simulink model "state_machine_by_code"  (R2021b)
settings: Solver=ode4  StartTime=0.0  StopTime=inf  FixedStep=0.001  RelTol=1e-3  EnableMultiTasking=on
model workspace (MATLAB code in the model file):
  | addpath src\model
  | addpath src\utils
libraries: rtlab x2
Description:
  | Model of a simple control system for use iin training.
settings Model: Creator=Paul Baracos  LastModifiedBy=andrerangel
settings SolverCC: AlgebraicLoopSolver=TrustRegion
settings DataIOCC: LimitDataPoints=on  SaveFormat=Array  SignalLoggingSaveFormat=ModelDataLogs  SaveOutput=off  SaveTime=off  ReturnWorkspaceOutputs=off  SignalLoggingName=sigsOut
settings OptimizationCC: BlockReduction=off  BooleanDataType=off  OptimizeBlockIOStorage=off  BufferReuse=off  ExpressionFolding=off  LocalBlockOutputs=off  InitFltsAndDblsToZero=on  LifeSpan=inf
settings DebuggingCC: SaveWithParameterizedLinksMsg=none  UnderspecifiedInitializationDetection=Classic  MergeDetectMultiDrivingBlocksExec=none  SignalResolutionControl=TryResolveAllWithWarning  MultiTaskDSMMsg=warning  MultiTaskCondExecSysMsg=none  FcnCallInpInsideContextMsg=warning  SFUnexpectedBacktrackingDiag=warning  SFNoUnconditionalDefaultTransitionDiag=warning  SFExecutionAtInitializationDiag=none  SFMachineParentedDataDiag=warning  ArithmeticOperatorsInVariantConditions=warning
settings HardwareCC: ProdBitPerPointer=32  ProdBitPerSizeT=32  ProdBitPerPtrDiffT=32  ProdLargestAtomicFloat=None  ProdIntDivRoundTo=Undefined  ProdEndianess=Unspecified  ProdWordSize=32  ProdHWDeviceType=32-bit Generic  TargetUnknown=on
settings ModelReferenceCC: PropagateSignalLabelsOutOfModel=off
settings SFSimCC: SimUseLocalCustomCode=off  CustomCodeUndefinedFunction=UseInterfaceOnly
settings RTWCC: RTWUseLocalCustomCode=off
settings CodeAppCC: StateflowObjectComments=on
settings GRTTargetCC: TargetFcnLib=ansi_tfl_tmw.mat  TargetLangStandard=C89/C90 (ANSI)  CombineOutputUpdateFcns=off  GRTInterface=on
settings ConfigComp: CovMetricSettings=dw  CovSaveCumulativeToWorkspaceVar=on  CovSaveSingleToWorkspaceVar=on  CovExternalEMLEnable=off

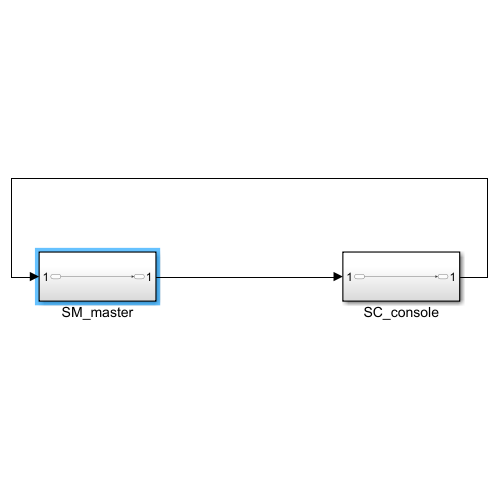
[thumbnail: Simulink's stored preview of the top-level diagram]
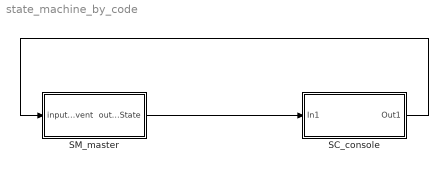
== system state_machine_by_code ==
  SC_console : Subsystem
  SM_master : Subsystem
  wires:
  SM_master/1(outputState) -> SC_console/1(In1)
  SC_console/1(Out1) -> SM_master/1(inputEvent)

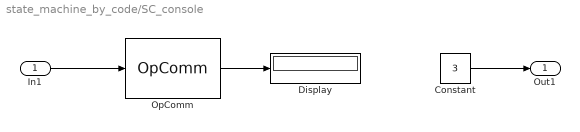
== system state_machine_by_code/SC_console ==
  In1 : Inport
  Constant : Constant  Value=3
  Display : Display
  OpComm : rtlab/OpComm  nbport=1  groupe_acq=1  subsys_rate=0  st=0  Synchronization=on  Interpolation=on  Threshold=1.0  Missed_Data=off  Sim_Time=off  Samples=off  dynSigOut=off  from_console=0  warning_done=off  writeOpCommFile=off  Offset=off
      settings: SourceProductName=RT-LAB
  Out1 : Outport
  wires:
  In1/1 -> OpComm/1
  Constant/1 -> Out1/1
  OpComm/1 -> Display/1

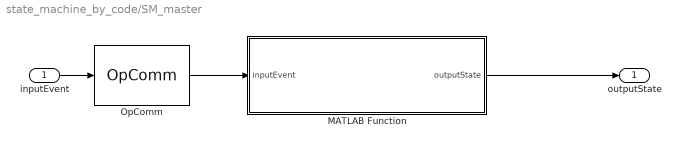
== system state_machine_by_code/SM_master ==
  inputEvent : Inport
  MATLAB Function : MATLAB Function  TreatAsAtomicUnit=on
  OpComm : rtlab/OpComm  nbport=1  groupe_acq=1  subsys_rate=0  st=0  Synchronization=on  Interpolation=on  Threshold=1.0  Missed_Data=off  Sim_Time=off  Samples=off  dynSigOut=off  from_console=1  warning_done=off  writeOpCommFile=off  Offset=off
      settings: SourceProductName=RT-LAB
  outputState : Outport
  wires:
  inputEvent/1 -> OpComm/1
  MATLAB Function/1(outputState) -> outputState/1
  OpComm/1 -> MATLAB Function/1(inputEvent)

== matlab function state_machine_by_code/SM_master/MATLAB Function ==
  data: inputEvent input; outputState output size=[1 1]
function outputState   = stateMachineFcn(inputEvent)
% Example of a State Machine with 3 states.
persistent stateMachine

if (isempty(stateMachine))
    
    % Create the states with the State Class.
    s0 = State(0, 's0', [1,0,1,1,1]);
    s1 = State(1, 's1', [1,1,0,1,1]);
    s2 = State(2, 's2', [1,0,1,1,1]);

    % Group it in a cell array.
    statesArray = {s0, s1, s2};

    % Transitions matrix where each line represents a transition: 
    % event 2 makes a transitions from state 0 to 2 is represented as 
    % [0 2 1]
    transitions = [0, 1 0; 0, 2, 1; 1, 3, 0; 1, 4, 2; 2, 5, 1; 2, 1, 0];

    % Array with the number of the events.
    eventsArray = [1 2 3 4 5];
    stateMachine = StateMachine(statesArray, transitions, eventsArray);
end

stateMachine.inputEvent = inputEvent;
outputState = double(stateMachine.currentState.number);

%activeEvents = stateMachine.currentState.activeEvents;
